simulink model "gm_MATE_HDLsolver_myFirstCircuit"  (R2024b)
settings: Solver=FixedStepDiscrete  StartTime=0.0  StopTime=0.05  FixedStep=6.02409638554217e-09  MaxStep=100e-6  RelTol=1e-4
PostLoadFcn:
  | Ts=1e-6; nb_sw=3; nb_lc=2;nb_r=1;nb_src=1; nb_out=3; rL=1.2;rC=100;L=1e-3; C=1e-5; LpejoSw=1e-6;h=Ts; MAX_INPUTS=16;
  | MAX_OUTPUTS=16;
  | MAX_SWITCHES=8;
  | MAX_INPUTS=16;
InitFcn:
  | Ts=1e-6; nb_sw=3; nb_lc=2;nb_r=1;nb_src=1; nb_out=3; rL=1.2;rC=100;L=1e-3; C=1e-5; LpejoSw=1e-6;h=Ts; MAX_INPUTS=16;
  | MAX_OUTPUTS=16;
  | MAX_SWITCHES=8;
  | MAX_INPUTS=16;
undefined symbols (not defined in the file or in its folder): MATE_SOC
libraries: fl_lib x31, nesl_utility x13, hdlmdlgenlib x10, simetranss x5, simulink x4, hdlsllib x3, ee_lib x2, eeGeneralControl x1
(part 4 of 8)

== system gm_MATE_HDLsolver_myFirstCircuit/ForFPGA/Dot Product1412 ==
  In1 : Inport
  In2 : Inport  Port=2
  Dot Product1412 : Sum  OutDataTypeStr=single  SampleTime=6.02409638554217e-09
  Dot Product1412_pd1 : Delay  DelayLength=6
  Out1 : Outport
  wires:
  In1/1 -> Dot Product1412/1
  In2/1 -> Dot Product1412/2
  Dot Product1412/1 -> Dot Product1412_pd1/1
  Dot Product1412_pd1/1 -> Out1/1

== system gm_MATE_HDLsolver_myFirstCircuit/ForFPGA/Dot Product1413 ==
  In1 : Inport
  In2 : Inport  Port=2
  Dot Product1413 : Sum  OutDataTypeStr=single  SampleTime=6.02409638554217e-09
  Dot Product1413_pd1 : Delay  DelayLength=6
  Out1 : Outport
  wires:
  In1/1 -> Dot Product1413/1
  In2/1 -> Dot Product1413/2
  Dot Product1413/1 -> Dot Product1413_pd1/1
  Dot Product1413_pd1/1 -> Out1/1

== system gm_MATE_HDLsolver_myFirstCircuit/ForFPGA/Dot Product1414 ==
  In1 : Inport
  In2 : Inport  Port=2
  Dot Product1414 : Sum  OutDataTypeStr=single  SampleTime=6.02409638554217e-09
  Dot Product1414_pd1 : Delay  DelayLength=6
  Out1 : Outport
  wires:
  In1/1 -> Dot Product1414/1
  In2/1 -> Dot Product1414/2
  Dot Product1414/1 -> Dot Product1414_pd1/1
  Dot Product1414_pd1/1 -> Out1/1

== system gm_MATE_HDLsolver_myFirstCircuit/ForFPGA/Dot Product1415 ==
  In1 : Inport
  In2 : Inport  Port=2
  Dot Product1415 : Sum  OutDataTypeStr=single  SampleTime=6.02409638554217e-09
  Dot Product1415_pd1 : Delay  DelayLength=6
  Out1 : Outport
  wires:
  In1/1 -> Dot Product1415/1
  In2/1 -> Dot Product1415/2
  Dot Product1415/1 -> Dot Product1415_pd1/1
  Dot Product1415_pd1/1 -> Out1/1

== system gm_MATE_HDLsolver_myFirstCircuit/ForFPGA/Dot Product142 ==
  In1 : Inport
  In2 : Inport  Port=2
  Dot Product142 : Sum  OutDataTypeStr=single  SampleTime=6.02409638554217e-09
  Dot Product142_pd1 : Delay  DelayLength=6
  Out1 : Outport
  wires:
  In1/1 -> Dot Product142/1
  In2/1 -> Dot Product142/2
  Dot Product142/1 -> Dot Product142_pd1/1
  Dot Product142_pd1/1 -> Out1/1

== system gm_MATE_HDLsolver_myFirstCircuit/ForFPGA/Dot Product143 ==
  In1 : Inport
  In2 : Inport  Port=2
  Dot Product143 : Sum  OutDataTypeStr=single  SampleTime=6.02409638554217e-09
  Dot Product143_pd1 : Delay  DelayLength=6
  Out1 : Outport
  wires:
  In1/1 -> Dot Product143/1
  In2/1 -> Dot Product143/2
  Dot Product143/1 -> Dot Product143_pd1/1
  Dot Product143_pd1/1 -> Out1/1

== system gm_MATE_HDLsolver_myFirstCircuit/ForFPGA/Dot Product144 ==
  In1 : Inport
  In2 : Inport  Port=2
  Dot Product144 : Sum  OutDataTypeStr=single  SampleTime=6.02409638554217e-09
  Dot Product144_pd1 : Delay  DelayLength=6
  Out1 : Outport
  wires:
  In1/1 -> Dot Product144/1
  In2/1 -> Dot Product144/2
  Dot Product144/1 -> Dot Product144_pd1/1
  Dot Product144_pd1/1 -> Out1/1

== system gm_MATE_HDLsolver_myFirstCircuit/ForFPGA/Dot Product145 ==
  In1 : Inport
  In2 : Inport  Port=2
  Dot Product145 : Sum  OutDataTypeStr=single  SampleTime=6.02409638554217e-09
  Dot Product145_pd1 : Delay  DelayLength=6
  Out1 : Outport
  wires:
  In1/1 -> Dot Product145/1
  In2/1 -> Dot Product145/2
  Dot Product145/1 -> Dot Product145_pd1/1
  Dot Product145_pd1/1 -> Out1/1

== system gm_MATE_HDLsolver_myFirstCircuit/ForFPGA/Dot Product146 ==
  In1 : Inport
  In2 : Inport  Port=2
  Dot Product146 : Sum  OutDataTypeStr=single  SampleTime=6.02409638554217e-09
  Dot Product146_pd1 : Delay  DelayLength=6
  Out1 : Outport
  wires:
  In1/1 -> Dot Product146/1
  In2/1 -> Dot Product146/2
  Dot Product146/1 -> Dot Product146_pd1/1
  Dot Product146_pd1/1 -> Out1/1

== system gm_MATE_HDLsolver_myFirstCircuit/ForFPGA/Dot Product147 ==
  In1 : Inport
  In2 : Inport  Port=2
  Dot Product147 : Sum  OutDataTypeStr=single  SampleTime=6.02409638554217e-09
  Dot Product147_pd1 : Delay  DelayLength=6
  Out1 : Outport
  wires:
  In1/1 -> Dot Product147/1
  In2/1 -> Dot Product147/2
  Dot Product147/1 -> Dot Product147_pd1/1
  Dot Product147_pd1/1 -> Out1/1

== system gm_MATE_HDLsolver_myFirstCircuit/ForFPGA/Dot Product148 ==
  In1 : Inport
  In2 : Inport  Port=2
  Dot Product148 : Sum  OutDataTypeStr=single  SampleTime=6.02409638554217e-09
  Dot Product148_pd1 : Delay  DelayLength=6
  Out1 : Outport
  wires:
  In1/1 -> Dot Product148/1
  In2/1 -> Dot Product148/2
  Dot Product148/1 -> Dot Product148_pd1/1
  Dot Product148_pd1/1 -> Out1/1

== system gm_MATE_HDLsolver_myFirstCircuit/ForFPGA/Dot Product149 ==
  In1 : Inport
  In2 : Inport  Port=2
  Dot Product149 : Sum  OutDataTypeStr=single  SampleTime=6.02409638554217e-09
  Dot Product149_pd1 : Delay  DelayLength=6
  Out1 : Outport
  wires:
  In1/1 -> Dot Product149/1
  In2/1 -> Dot Product149/2
  Dot Product149/1 -> Dot Product149_pd1/1
  Dot Product149_pd1/1 -> Out1/1

== system gm_MATE_HDLsolver_myFirstCircuit/ForFPGA/Dot Product15 ==
  In1 : Inport
  In2 : Inport  Port=2
  Dot Product15 : Sum  OutDataTypeStr=single  SampleTime=6.02409638554217e-09
  Dot Product15_pd1 : Delay  DelayLength=6
  Out1 : Outport
  wires:
  In1/1 -> Dot Product15/1
  In2/1 -> Dot Product15/2
  Dot Product15/1 -> Dot Product15_pd1/1
  Dot Product15_pd1/1 -> Out1/1

== system gm_MATE_HDLsolver_myFirstCircuit/ForFPGA/Dot Product151 ==
  In1 : Inport
  In2 : Inport  Port=2
  Dot Product151 : Sum  OutDataTypeStr=single  SampleTime=6.02409638554217e-09
  Dot Product151_pd1 : Delay  DelayLength=6
  Out1 : Outport
  wires:
  In1/1 -> Dot Product151/1
  In2/1 -> Dot Product151/2
  Dot Product151/1 -> Dot Product151_pd1/1
  Dot Product151_pd1/1 -> Out1/1

== system gm_MATE_HDLsolver_myFirstCircuit/ForFPGA/Dot Product1510 ==
  In1 : Inport
  In2 : Inport  Port=2
  Dot Product1510 : Sum  OutDataTypeStr=single  SampleTime=6.02409638554217e-09
  Dot Product1510_pd1 : Delay  DelayLength=6
  Out1 : Outport
  wires:
  In1/1 -> Dot Product1510/1
  In2/1 -> Dot Product1510/2
  Dot Product1510/1 -> Dot Product1510_pd1/1
  Dot Product1510_pd1/1 -> Out1/1

== system gm_MATE_HDLsolver_myFirstCircuit/ForFPGA/Dot Product1511 ==
  In1 : Inport
  In2 : Inport  Port=2
  Dot Product1511 : Sum  OutDataTypeStr=single  SampleTime=6.02409638554217e-09
  Dot Product1511_pd1 : Delay  DelayLength=6
  Out1 : Outport
  wires:
  In1/1 -> Dot Product1511/1
  In2/1 -> Dot Product1511/2
  Dot Product1511/1 -> Dot Product1511_pd1/1
  Dot Product1511_pd1/1 -> Out1/1

== system gm_MATE_HDLsolver_myFirstCircuit/ForFPGA/Dot Product1512 ==
  In1 : Inport
  In2 : Inport  Port=2
  Dot Product1512 : Sum  OutDataTypeStr=single  SampleTime=6.02409638554217e-09
  Dot Product1512_pd1 : Delay  DelayLength=6
  Out1 : Outport
  wires:
  In1/1 -> Dot Product1512/1
  In2/1 -> Dot Product1512/2
  Dot Product1512/1 -> Dot Product1512_pd1/1
  Dot Product1512_pd1/1 -> Out1/1

== system gm_MATE_HDLsolver_myFirstCircuit/ForFPGA/Dot Product1513 ==
  In1 : Inport
  In2 : Inport  Port=2
  Dot Product1513 : Sum  OutDataTypeStr=single  SampleTime=6.02409638554217e-09
  Dot Product1513_pd1 : Delay  DelayLength=6
  Out1 : Outport
  wires:
  In1/1 -> Dot Product1513/1
  In2/1 -> Dot Product1513/2
  Dot Product1513/1 -> Dot Product1513_pd1/1
  Dot Product1513_pd1/1 -> Out1/1

== system gm_MATE_HDLsolver_myFirstCircuit/ForFPGA/Dot Product1514 ==
  In1 : Inport
  In2 : Inport  Port=2
  Dot Product1514 : Sum  OutDataTypeStr=single  SampleTime=6.02409638554217e-09
  Dot Product1514_pd1 : Delay  DelayLength=6
  Out1 : Outport
  wires:
  In1/1 -> Dot Product1514/1
  In2/1 -> Dot Product1514/2
  Dot Product1514/1 -> Dot Product1514_pd1/1
  Dot Product1514_pd1/1 -> Out1/1

== system gm_MATE_HDLsolver_myFirstCircuit/ForFPGA/Dot Product1515 ==
  In1 : Inport
  In2 : Inport  Port=2
  Dot Product1515 : Sum  OutDataTypeStr=single  SampleTime=6.02409638554217e-09
  Dot Product1515_pd1 : Delay  DelayLength=6
  Out1 : Outport
  wires:
  In1/1 -> Dot Product1515/1
  In2/1 -> Dot Product1515/2
  Dot Product1515/1 -> Dot Product1515_pd1/1
  Dot Product1515_pd1/1 -> Out1/1

== system gm_MATE_HDLsolver_myFirstCircuit/ForFPGA/Dot Product152 ==
  In1 : Inport
  In2 : Inport  Port=2
  Dot Product152 : Sum  OutDataTypeStr=single  SampleTime=6.02409638554217e-09
  Dot Product152_pd1 : Delay  DelayLength=6
  Out1 : Outport
  wires:
  In1/1 -> Dot Product152/1
  In2/1 -> Dot Product152/2
  Dot Product152/1 -> Dot Product152_pd1/1
  Dot Product152_pd1/1 -> Out1/1

== system gm_MATE_HDLsolver_myFirstCircuit/ForFPGA/Dot Product153 ==
  In1 : Inport
  In2 : Inport  Port=2
  Dot Product153 : Sum  OutDataTypeStr=single  SampleTime=6.02409638554217e-09
  Dot Product153_pd1 : Delay  DelayLength=6
  Out1 : Outport
  wires:
  In1/1 -> Dot Product153/1
  In2/1 -> Dot Product153/2
  Dot Product153/1 -> Dot Product153_pd1/1
  Dot Product153_pd1/1 -> Out1/1

== system gm_MATE_HDLsolver_myFirstCircuit/ForFPGA/Dot Product154 ==
  In1 : Inport
  In2 : Inport  Port=2
  Dot Product154 : Sum  OutDataTypeStr=single  SampleTime=6.02409638554217e-09
  Dot Product154_pd1 : Delay  DelayLength=6
  Out1 : Outport
  wires:
  In1/1 -> Dot Product154/1
  In2/1 -> Dot Product154/2
  Dot Product154/1 -> Dot Product154_pd1/1
  Dot Product154_pd1/1 -> Out1/1

== system gm_MATE_HDLsolver_myFirstCircuit/ForFPGA/Dot Product155 ==
  In1 : Inport
  In2 : Inport  Port=2
  Dot Product155 : Sum  OutDataTypeStr=single  SampleTime=6.02409638554217e-09
  Dot Product155_pd1 : Delay  DelayLength=6
  Out1 : Outport
  wires:
  In1/1 -> Dot Product155/1
  In2/1 -> Dot Product155/2
  Dot Product155/1 -> Dot Product155_pd1/1
  Dot Product155_pd1/1 -> Out1/1

== system gm_MATE_HDLsolver_myFirstCircuit/ForFPGA/Dot Product156 ==
  In1 : Inport
  In2 : Inport  Port=2
  Dot Product156 : Sum  OutDataTypeStr=single  SampleTime=6.02409638554217e-09
  Dot Product156_pd1 : Delay  DelayLength=6
  Out1 : Outport
  wires:
  In1/1 -> Dot Product156/1
  In2/1 -> Dot Product156/2
  Dot Product156/1 -> Dot Product156_pd1/1
  Dot Product156_pd1/1 -> Out1/1

== system gm_MATE_HDLsolver_myFirstCircuit/ForFPGA/Dot Product157 ==
  In1 : Inport
  In2 : Inport  Port=2
  Dot Product157 : Sum  OutDataTypeStr=single  SampleTime=6.02409638554217e-09
  Dot Product157_pd1 : Delay  DelayLength=6
  Out1 : Outport
  wires:
  In1/1 -> Dot Product157/1
  In2/1 -> Dot Product157/2
  Dot Product157/1 -> Dot Product157_pd1/1
  Dot Product157_pd1/1 -> Out1/1

== system gm_MATE_HDLsolver_myFirstCircuit/ForFPGA/Dot Product158 ==
  In1 : Inport
  In2 : Inport  Port=2
  Dot Product158 : Sum  OutDataTypeStr=single  SampleTime=6.02409638554217e-09
  Dot Product158_pd1 : Delay  DelayLength=6
  Out1 : Outport
  wires:
  In1/1 -> Dot Product158/1
  In2/1 -> Dot Product158/2
  Dot Product158/1 -> Dot Product158_pd1/1
  Dot Product158_pd1/1 -> Out1/1

== system gm_MATE_HDLsolver_myFirstCircuit/ForFPGA/Dot Product159 ==
  In1 : Inport
  In2 : Inport  Port=2
  Dot Product159 : Sum  OutDataTypeStr=single  SampleTime=6.02409638554217e-09
  Dot Product159_pd1 : Delay  DelayLength=6
  Out1 : Outport
  wires:
  In1/1 -> Dot Product159/1
  In2/1 -> Dot Product159/2
  Dot Product159/1 -> Dot Product159_pd1/1
  Dot Product159_pd1/1 -> Out1/1

== system gm_MATE_HDLsolver_myFirstCircuit/ForFPGA/Dot Product16 ==
  In1 : Inport
  In2 : Inport  Port=2
  Dot Product16 : Sum  OutDataTypeStr=single  SampleTime=6.02409638554217e-09
  Dot Product16_pd1 : Delay  DelayLength=6
  Out1 : Outport
  wires:
  In1/1 -> Dot Product16/1
  In2/1 -> Dot Product16/2
  Dot Product16/1 -> Dot Product16_pd1/1
  Dot Product16_pd1/1 -> Out1/1

== system gm_MATE_HDLsolver_myFirstCircuit/ForFPGA/Dot Product17 ==
  In1 : Inport
  In2 : Inport  Port=2
  Dot Product17 : Sum  OutDataTypeStr=single  SampleTime=6.02409638554217e-09
  Dot Product17_pd1 : Delay  DelayLength=6
  Out1 : Outport
  wires:
  In1/1 -> Dot Product17/1
  In2/1 -> Dot Product17/2
  Dot Product17/1 -> Dot Product17_pd1/1
  Dot Product17_pd1/1 -> Out1/1

== system gm_MATE_HDLsolver_myFirstCircuit/ForFPGA/Dot Product18 ==
  In1 : Inport
  In2 : Inport  Port=2
  Dot Product18 : Sum  OutDataTypeStr=single  SampleTime=6.02409638554217e-09
  Dot Product18_pd1 : Delay  DelayLength=6
  Out1 : Outport
  wires:
  In1/1 -> Dot Product18/1
  In2/1 -> Dot Product18/2
  Dot Product18/1 -> Dot Product18_pd1/1
  Dot Product18_pd1/1 -> Out1/1

== system gm_MATE_HDLsolver_myFirstCircuit/ForFPGA/Dot Product19 ==
  In1 : Inport
  In2 : Inport  Port=2
  Dot Product19 : Sum  OutDataTypeStr=single  SampleTime=6.02409638554217e-09
  Dot Product19_pd1 : Delay  DelayLength=6
  Out1 : Outport
  wires:
  In1/1 -> Dot Product19/1
  In2/1 -> Dot Product19/2
  Dot Product19/1 -> Dot Product19_pd1/1
  Dot Product19_pd1/1 -> Out1/1

== system gm_MATE_HDLsolver_myFirstCircuit/ForFPGA/Dot Product2 ==
  In1 : Inport
  In2 : Inport  Port=2
  Dot Product2 : Sum  OutDataTypeStr=single  SampleTime=6.02409638554217e-09
  Dot Product2_pd1 : Delay  DelayLength=6
  Out1 : Outport
  wires:
  In1/1 -> Dot Product2/1
  In2/1 -> Dot Product2/2
  Dot Product2/1 -> Dot Product2_pd1/1
  Dot Product2_pd1/1 -> Out1/1

== system gm_MATE_HDLsolver_myFirstCircuit/ForFPGA/Dot Product21 ==
  In1 : Inport
  In2 : Inport  Port=2
  Dot Product21 : Sum  OutDataTypeStr=single  SampleTime=6.02409638554217e-09
  Dot Product21_pd1 : Delay  DelayLength=6
  Out1 : Outport
  wires:
  In1/1 -> Dot Product21/1
  In2/1 -> Dot Product21/2
  Dot Product21/1 -> Dot Product21_pd1/1
  Dot Product21_pd1/1 -> Out1/1

== system gm_MATE_HDLsolver_myFirstCircuit/ForFPGA/Dot Product210 ==
  In1 : Inport
  In2 : Inport  Port=2
  Dot Product210 : Sum  OutDataTypeStr=single  SampleTime=6.02409638554217e-09
  Dot Product210_pd1 : Delay  DelayLength=6
  Out1 : Outport
  wires:
  In1/1 -> Dot Product210/1
  In2/1 -> Dot Product210/2
  Dot Product210/1 -> Dot Product210_pd1/1
  Dot Product210_pd1/1 -> Out1/1

== system gm_MATE_HDLsolver_myFirstCircuit/ForFPGA/Dot Product211 ==
  In1 : Inport
  In2 : Inport  Port=2
  Dot Product211 : Sum  OutDataTypeStr=single  SampleTime=6.02409638554217e-09
  Dot Product211_pd1 : Delay  DelayLength=6
  Out1 : Outport
  wires:
  In1/1 -> Dot Product211/1
  In2/1 -> Dot Product211/2
  Dot Product211/1 -> Dot Product211_pd1/1
  Dot Product211_pd1/1 -> Out1/1

== system gm_MATE_HDLsolver_myFirstCircuit/ForFPGA/Dot Product212 ==
  In1 : Inport
  In2 : Inport  Port=2
  Dot Product212 : Sum  OutDataTypeStr=single  SampleTime=6.02409638554217e-09
  Dot Product212_pd1 : Delay  DelayLength=6
  Out1 : Outport
  wires:
  In1/1 -> Dot Product212/1
  In2/1 -> Dot Product212/2
  Dot Product212/1 -> Dot Product212_pd1/1
  Dot Product212_pd1/1 -> Out1/1

== system gm_MATE_HDLsolver_myFirstCircuit/ForFPGA/Dot Product213 ==
  In1 : Inport
  In2 : Inport  Port=2
  Dot Product213 : Sum  OutDataTypeStr=single  SampleTime=6.02409638554217e-09
  Dot Product213_pd1 : Delay  DelayLength=6
  Out1 : Outport
  wires:
  In1/1 -> Dot Product213/1
  In2/1 -> Dot Product213/2
  Dot Product213/1 -> Dot Product213_pd1/1
  Dot Product213_pd1/1 -> Out1/1

== system gm_MATE_HDLsolver_myFirstCircuit/ForFPGA/Dot Product214 ==
  In1 : Inport
  In2 : Inport  Port=2
  Dot Product214 : Sum  OutDataTypeStr=single  SampleTime=6.02409638554217e-09
  Dot Product214_pd1 : Delay  DelayLength=6
  Out1 : Outport
  wires:
  In1/1 -> Dot Product214/1
  In2/1 -> Dot Product214/2
  Dot Product214/1 -> Dot Product214_pd1/1
  Dot Product214_pd1/1 -> Out1/1

== system gm_MATE_HDLsolver_myFirstCircuit/ForFPGA/Dot Product215 ==
  In1 : Inport
  In2 : Inport  Port=2
  Dot Product215 : Sum  OutDataTypeStr=single  SampleTime=6.02409638554217e-09
  Dot Product215_pd1 : Delay  DelayLength=6
  Out1 : Outport
  wires:
  In1/1 -> Dot Product215/1
  In2/1 -> Dot Product215/2
  Dot Product215/1 -> Dot Product215_pd1/1
  Dot Product215_pd1/1 -> Out1/1

== system gm_MATE_HDLsolver_myFirstCircuit/ForFPGA/Dot Product22 ==
  In1 : Inport
  In2 : Inport  Port=2
  Dot Product22 : Sum  OutDataTypeStr=single  SampleTime=6.02409638554217e-09
  Dot Product22_pd1 : Delay  DelayLength=6
  Out1 : Outport
  wires:
  In1/1 -> Dot Product22/1
  In2/1 -> Dot Product22/2
  Dot Product22/1 -> Dot Product22_pd1/1
  Dot Product22_pd1/1 -> Out1/1

== system gm_MATE_HDLsolver_myFirstCircuit/ForFPGA/Dot Product23 ==
  In1 : Inport
  In2 : Inport  Port=2
  Dot Product23 : Sum  OutDataTypeStr=single  SampleTime=6.02409638554217e-09
  Dot Product23_pd1 : Delay  DelayLength=6
  Out1 : Outport
  wires:
  In1/1 -> Dot Product23/1
  In2/1 -> Dot Product23/2
  Dot Product23/1 -> Dot Product23_pd1/1
  Dot Product23_pd1/1 -> Out1/1

== system gm_MATE_HDLsolver_myFirstCircuit/ForFPGA/Dot Product24 ==
  In1 : Inport
  In2 : Inport  Port=2
  Dot Product24 : Sum  OutDataTypeStr=single  SampleTime=6.02409638554217e-09
  Dot Product24_pd1 : Delay  DelayLength=6
  Out1 : Outport
  wires:
  In1/1 -> Dot Product24/1
  In2/1 -> Dot Product24/2
  Dot Product24/1 -> Dot Product24_pd1/1
  Dot Product24_pd1/1 -> Out1/1

== system gm_MATE_HDLsolver_myFirstCircuit/ForFPGA/Dot Product25 ==
  In1 : Inport
  In2 : Inport  Port=2
  Dot Product25 : Sum  OutDataTypeStr=single  SampleTime=6.02409638554217e-09
  Dot Product25_pd1 : Delay  DelayLength=6
  Out1 : Outport
  wires:
  In1/1 -> Dot Product25/1
  In2/1 -> Dot Product25/2
  Dot Product25/1 -> Dot Product25_pd1/1
  Dot Product25_pd1/1 -> Out1/1

== system gm_MATE_HDLsolver_myFirstCircuit/ForFPGA/Dot Product26 ==
  In1 : Inport
  In2 : Inport  Port=2
  Dot Product26 : Sum  OutDataTypeStr=single  SampleTime=6.02409638554217e-09
  Dot Product26_pd1 : Delay  DelayLength=6
  Out1 : Outport
  wires:
  In1/1 -> Dot Product26/1
  In2/1 -> Dot Product26/2
  Dot Product26/1 -> Dot Product26_pd1/1
  Dot Product26_pd1/1 -> Out1/1

== system gm_MATE_HDLsolver_myFirstCircuit/ForFPGA/Dot Product27 ==
  In1 : Inport
  In2 : Inport  Port=2
  Dot Product27 : Sum  OutDataTypeStr=single  SampleTime=6.02409638554217e-09
  Dot Product27_pd1 : Delay  DelayLength=6
  Out1 : Outport
  wires:
  In1/1 -> Dot Product27/1
  In2/1 -> Dot Product27/2
  Dot Product27/1 -> Dot Product27_pd1/1
  Dot Product27_pd1/1 -> Out1/1

== system gm_MATE_HDLsolver_myFirstCircuit/ForFPGA/Dot Product28 ==
  In1 : Inport
  In2 : Inport  Port=2
  Dot Product28 : Sum  OutDataTypeStr=single  SampleTime=6.02409638554217e-09
  Dot Product28_pd1 : Delay  DelayLength=6
  Out1 : Outport
  wires:
  In1/1 -> Dot Product28/1
  In2/1 -> Dot Product28/2
  Dot Product28/1 -> Dot Product28_pd1/1
  Dot Product28_pd1/1 -> Out1/1

== system gm_MATE_HDLsolver_myFirstCircuit/ForFPGA/Dot Product29 ==
  In1 : Inport
  In2 : Inport  Port=2
  Dot Product29 : Sum  OutDataTypeStr=single  SampleTime=6.02409638554217e-09
  Dot Product29_pd1 : Delay  DelayLength=6
  Out1 : Outport
  wires:
  In1/1 -> Dot Product29/1
  In2/1 -> Dot Product29/2
  Dot Product29/1 -> Dot Product29_pd1/1
  Dot Product29_pd1/1 -> Out1/1

== system gm_MATE_HDLsolver_myFirstCircuit/ForFPGA/Dot Product3 ==
  In1 : Inport
  In2 : Inport  Port=2
  Dot Product3 : Sum  OutDataTypeStr=single  SampleTime=6.02409638554217e-09
  Dot Product3_pd1 : Delay  DelayLength=6
  Out1 : Outport
  wires:
  In1/1 -> Dot Product3/1
  In2/1 -> Dot Product3/2
  Dot Product3/1 -> Dot Product3_pd1/1
  Dot Product3_pd1/1 -> Out1/1

== system gm_MATE_HDLsolver_myFirstCircuit/ForFPGA/Dot Product31 ==
  In1 : Inport
  In2 : Inport  Port=2
  Dot Product31 : Sum  OutDataTypeStr=single  SampleTime=6.02409638554217e-09
  Dot Product31_pd1 : Delay  DelayLength=6
  Out1 : Outport
  wires:
  In1/1 -> Dot Product31/1
  In2/1 -> Dot Product31/2
  Dot Product31/1 -> Dot Product31_pd1/1
  Dot Product31_pd1/1 -> Out1/1

== system gm_MATE_HDLsolver_myFirstCircuit/ForFPGA/Dot Product310 ==
  In1 : Inport
  In2 : Inport  Port=2
  Dot Product310 : Sum  OutDataTypeStr=single  SampleTime=6.02409638554217e-09
  Dot Product310_pd1 : Delay  DelayLength=6
  Out1 : Outport
  wires:
  In1/1 -> Dot Product310/1
  In2/1 -> Dot Product310/2
  Dot Product310/1 -> Dot Product310_pd1/1
  Dot Product310_pd1/1 -> Out1/1

== system gm_MATE_HDLsolver_myFirstCircuit/ForFPGA/Dot Product311 ==
  In1 : Inport
  In2 : Inport  Port=2
  Dot Product311 : Sum  OutDataTypeStr=single  SampleTime=6.02409638554217e-09
  Dot Product311_pd1 : Delay  DelayLength=6
  Out1 : Outport
  wires:
  In1/1 -> Dot Product311/1
  In2/1 -> Dot Product311/2
  Dot Product311/1 -> Dot Product311_pd1/1
  Dot Product311_pd1/1 -> Out1/1

== system gm_MATE_HDLsolver_myFirstCircuit/ForFPGA/Dot Product312 ==
  In1 : Inport
  In2 : Inport  Port=2
  Dot Product312 : Sum  OutDataTypeStr=single  SampleTime=6.02409638554217e-09
  Dot Product312_pd1 : Delay  DelayLength=6
  Out1 : Outport
  wires:
  In1/1 -> Dot Product312/1
  In2/1 -> Dot Product312/2
  Dot Product312/1 -> Dot Product312_pd1/1
  Dot Product312_pd1/1 -> Out1/1

== system gm_MATE_HDLsolver_myFirstCircuit/ForFPGA/Dot Product313 ==
  In1 : Inport
  In2 : Inport  Port=2
  Dot Product313 : Sum  OutDataTypeStr=single  SampleTime=6.02409638554217e-09
  Dot Product313_pd1 : Delay  DelayLength=6
  Out1 : Outport
  wires:
  In1/1 -> Dot Product313/1
  In2/1 -> Dot Product313/2
  Dot Product313/1 -> Dot Product313_pd1/1
  Dot Product313_pd1/1 -> Out1/1

== system gm_MATE_HDLsolver_myFirstCircuit/ForFPGA/Dot Product314 ==
  In1 : Inport
  In2 : Inport  Port=2
  Dot Product314 : Sum  OutDataTypeStr=single  SampleTime=6.02409638554217e-09
  Dot Product314_pd1 : Delay  DelayLength=6
  Out1 : Outport
  wires:
  In1/1 -> Dot Product314/1
  In2/1 -> Dot Product314/2
  Dot Product314/1 -> Dot Product314_pd1/1
  Dot Product314_pd1/1 -> Out1/1

== system gm_MATE_HDLsolver_myFirstCircuit/ForFPGA/Dot Product315 ==
  In1 : Inport
  In2 : Inport  Port=2
  Dot Product315 : Sum  OutDataTypeStr=single  SampleTime=6.02409638554217e-09
  Dot Product315_pd1 : Delay  DelayLength=6
  Out1 : Outport
  wires:
  In1/1 -> Dot Product315/1
  In2/1 -> Dot Product315/2
  Dot Product315/1 -> Dot Product315_pd1/1
  Dot Product315_pd1/1 -> Out1/1

== system gm_MATE_HDLsolver_myFirstCircuit/ForFPGA/Dot Product32 ==
  In1 : Inport
  In2 : Inport  Port=2
  Dot Product32 : Sum  OutDataTypeStr=single  SampleTime=6.02409638554217e-09
  Dot Product32_pd1 : Delay  DelayLength=6
  Out1 : Outport
  wires:
  In1/1 -> Dot Product32/1
  In2/1 -> Dot Product32/2
  Dot Product32/1 -> Dot Product32_pd1/1
  Dot Product32_pd1/1 -> Out1/1

== system gm_MATE_HDLsolver_myFirstCircuit/ForFPGA/Dot Product33 ==
  In1 : Inport
  In2 : Inport  Port=2
  Dot Product33 : Sum  OutDataTypeStr=single  SampleTime=6.02409638554217e-09
  Dot Product33_pd1 : Delay  DelayLength=6
  Out1 : Outport
  wires:
  In1/1 -> Dot Product33/1
  In2/1 -> Dot Product33/2
  Dot Product33/1 -> Dot Product33_pd1/1
  Dot Product33_pd1/1 -> Out1/1

== system gm_MATE_HDLsolver_myFirstCircuit/ForFPGA/Dot Product34 ==
  In1 : Inport
  In2 : Inport  Port=2
  Dot Product34 : Sum  OutDataTypeStr=single  SampleTime=6.02409638554217e-09
  Dot Product34_pd1 : Delay  DelayLength=6
  Out1 : Outport
  wires:
  In1/1 -> Dot Product34/1
  In2/1 -> Dot Product34/2
  Dot Product34/1 -> Dot Product34_pd1/1
  Dot Product34_pd1/1 -> Out1/1

== system gm_MATE_HDLsolver_myFirstCircuit/ForFPGA/Dot Product35 ==
  In1 : Inport
  In2 : Inport  Port=2
  Dot Product35 : Sum  OutDataTypeStr=single  SampleTime=6.02409638554217e-09
  Dot Product35_pd1 : Delay  DelayLength=6
  Out1 : Outport
  wires:
  In1/1 -> Dot Product35/1
  In2/1 -> Dot Product35/2
  Dot Product35/1 -> Dot Product35_pd1/1
  Dot Product35_pd1/1 -> Out1/1

== system gm_MATE_HDLsolver_myFirstCircuit/ForFPGA/Dot Product36 ==
  In1 : Inport
  In2 : Inport  Port=2
  Dot Product36 : Sum  OutDataTypeStr=single  SampleTime=6.02409638554217e-09
  Dot Product36_pd1 : Delay  DelayLength=6
  Out1 : Outport
  wires:
  In1/1 -> Dot Product36/1
  In2/1 -> Dot Product36/2
  Dot Product36/1 -> Dot Product36_pd1/1
  Dot Product36_pd1/1 -> Out1/1

== system gm_MATE_HDLsolver_myFirstCircuit/ForFPGA/Dot Product37 ==
  In1 : Inport
  In2 : Inport  Port=2
  Dot Product37 : Sum  OutDataTypeStr=single  SampleTime=6.02409638554217e-09
  Dot Product37_pd1 : Delay  DelayLength=6
  Out1 : Outport
  wires:
  In1/1 -> Dot Product37/1
  In2/1 -> Dot Product37/2
  Dot Product37/1 -> Dot Product37_pd1/1
  Dot Product37_pd1/1 -> Out1/1

== system gm_MATE_HDLsolver_myFirstCircuit/ForFPGA/Dot Product38 ==
  In1 : Inport
  In2 : Inport  Port=2
  Dot Product38 : Sum  OutDataTypeStr=single  SampleTime=6.02409638554217e-09
  Dot Product38_pd1 : Delay  DelayLength=6
  Out1 : Outport
  wires:
  In1/1 -> Dot Product38/1
  In2/1 -> Dot Product38/2
  Dot Product38/1 -> Dot Product38_pd1/1
  Dot Product38_pd1/1 -> Out1/1

== system gm_MATE_HDLsolver_myFirstCircuit/ForFPGA/Dot Product39 ==
  In1 : Inport
  In2 : Inport  Port=2
  Dot Product39 : Sum  OutDataTypeStr=single  SampleTime=6.02409638554217e-09
  Dot Product39_pd1 : Delay  DelayLength=6
  Out1 : Outport
  wires:
  In1/1 -> Dot Product39/1
  In2/1 -> Dot Product39/2
  Dot Product39/1 -> Dot Product39_pd1/1
  Dot Product39_pd1/1 -> Out1/1

== system gm_MATE_HDLsolver_myFirstCircuit/ForFPGA/Dot Product4 ==
  In1 : Inport
  In2 : Inport  Port=2
  Dot Product4 : Sum  OutDataTypeStr=single  SampleTime=6.02409638554217e-09
  Dot Product4_pd1 : Delay  DelayLength=6
  Out1 : Outport
  wires:
  In1/1 -> Dot Product4/1
  In2/1 -> Dot Product4/2
  Dot Product4/1 -> Dot Product4_pd1/1
  Dot Product4_pd1/1 -> Out1/1

== system gm_MATE_HDLsolver_myFirstCircuit/ForFPGA/Dot Product41 ==
  In1 : Inport
  In2 : Inport  Port=2
  Dot Product41 : Sum  OutDataTypeStr=single  SampleTime=6.02409638554217e-09
  Dot Product41_pd1 : Delay  DelayLength=6
  Out1 : Outport
  wires:
  In1/1 -> Dot Product41/1
  In2/1 -> Dot Product41/2
  Dot Product41/1 -> Dot Product41_pd1/1
  Dot Product41_pd1/1 -> Out1/1

== system gm_MATE_HDLsolver_myFirstCircuit/ForFPGA/Dot Product410 ==
  In1 : Inport
  In2 : Inport  Port=2
  Dot Product410 : Sum  OutDataTypeStr=single  SampleTime=6.02409638554217e-09
  Dot Product410_pd1 : Delay  DelayLength=6
  Out1 : Outport
  wires:
  In1/1 -> Dot Product410/1
  In2/1 -> Dot Product410/2
  Dot Product410/1 -> Dot Product410_pd1/1
  Dot Product410_pd1/1 -> Out1/1

== system gm_MATE_HDLsolver_myFirstCircuit/ForFPGA/Dot Product411 ==
  In1 : Inport
  In2 : Inport  Port=2
  Dot Product411 : Sum  OutDataTypeStr=single  SampleTime=6.02409638554217e-09
  Dot Product411_pd1 : Delay  DelayLength=6
  Out1 : Outport
  wires:
  In1/1 -> Dot Product411/1
  In2/1 -> Dot Product411/2
  Dot Product411/1 -> Dot Product411_pd1/1
  Dot Product411_pd1/1 -> Out1/1

== system gm_MATE_HDLsolver_myFirstCircuit/ForFPGA/Dot Product412 ==
  In1 : Inport
  In2 : Inport  Port=2
  Dot Product412 : Sum  OutDataTypeStr=single  SampleTime=6.02409638554217e-09
  Dot Product412_pd1 : Delay  DelayLength=6
  Out1 : Outport
  wires:
  In1/1 -> Dot Product412/1
  In2/1 -> Dot Product412/2
  Dot Product412/1 -> Dot Product412_pd1/1
  Dot Product412_pd1/1 -> Out1/1

== system gm_MATE_HDLsolver_myFirstCircuit/ForFPGA/Dot Product413 ==
  In1 : Inport
  In2 : Inport  Port=2
  Dot Product413 : Sum  OutDataTypeStr=single  SampleTime=6.02409638554217e-09
  Dot Product413_pd1 : Delay  DelayLength=6
  Out1 : Outport
  wires:
  In1/1 -> Dot Product413/1
  In2/1 -> Dot Product413/2
  Dot Product413/1 -> Dot Product413_pd1/1
  Dot Product413_pd1/1 -> Out1/1

== system gm_MATE_HDLsolver_myFirstCircuit/ForFPGA/Dot Product414 ==
  In1 : Inport
  In2 : Inport  Port=2
  Dot Product414 : Sum  OutDataTypeStr=single  SampleTime=6.02409638554217e-09
  Dot Product414_pd1 : Delay  DelayLength=6
  Out1 : Outport
  wires:
  In1/1 -> Dot Product414/1
  In2/1 -> Dot Product414/2
  Dot Product414/1 -> Dot Product414_pd1/1
  Dot Product414_pd1/1 -> Out1/1

== system gm_MATE_HDLsolver_myFirstCircuit/ForFPGA/Dot Product415 ==
  In1 : Inport
  In2 : Inport  Port=2
  Dot Product415 : Sum  OutDataTypeStr=single  SampleTime=6.02409638554217e-09
  Dot Product415_pd1 : Delay  DelayLength=6
  Out1 : Outport
  wires:
  In1/1 -> Dot Product415/1
  In2/1 -> Dot Product415/2
  Dot Product415/1 -> Dot Product415_pd1/1
  Dot Product415_pd1/1 -> Out1/1

== system gm_MATE_HDLsolver_myFirstCircuit/ForFPGA/Dot Product42 ==
  In1 : Inport
  In2 : Inport  Port=2
  Dot Product42 : Sum  OutDataTypeStr=single  SampleTime=6.02409638554217e-09
  Dot Product42_pd1 : Delay  DelayLength=6
  Out1 : Outport
  wires:
  In1/1 -> Dot Product42/1
  In2/1 -> Dot Product42/2
  Dot Product42/1 -> Dot Product42_pd1/1
  Dot Product42_pd1/1 -> Out1/1

== system gm_MATE_HDLsolver_myFirstCircuit/ForFPGA/Dot Product43 ==
  In1 : Inport
  In2 : Inport  Port=2
  Dot Product43 : Sum  OutDataTypeStr=single  SampleTime=6.02409638554217e-09
  Dot Product43_pd1 : Delay  DelayLength=6
  Out1 : Outport
  wires:
  In1/1 -> Dot Product43/1
  In2/1 -> Dot Product43/2
  Dot Product43/1 -> Dot Product43_pd1/1
  Dot Product43_pd1/1 -> Out1/1

== system gm_MATE_HDLsolver_myFirstCircuit/ForFPGA/Dot Product44 ==
  In1 : Inport
  In2 : Inport  Port=2
  Dot Product44 : Sum  OutDataTypeStr=single  SampleTime=6.02409638554217e-09
  Dot Product44_pd1 : Delay  DelayLength=6
  Out1 : Outport
  wires:
  In1/1 -> Dot Product44/1
  In2/1 -> Dot Product44/2
  Dot Product44/1 -> Dot Product44_pd1/1
  Dot Product44_pd1/1 -> Out1/1

== system gm_MATE_HDLsolver_myFirstCircuit/ForFPGA/Dot Product45 ==
  In1 : Inport
  In2 : Inport  Port=2
  Dot Product45 : Sum  OutDataTypeStr=single  SampleTime=6.02409638554217e-09
  Dot Product45_pd1 : Delay  DelayLength=6
  Out1 : Outport
  wires:
  In1/1 -> Dot Product45/1
  In2/1 -> Dot Product45/2
  Dot Product45/1 -> Dot Product45_pd1/1
  Dot Product45_pd1/1 -> Out1/1

== system gm_MATE_HDLsolver_myFirstCircuit/ForFPGA/Dot Product46 ==
  In1 : Inport
  In2 : Inport  Port=2
  Dot Product46 : Sum  OutDataTypeStr=single  SampleTime=6.02409638554217e-09
  Dot Product46_pd1 : Delay  DelayLength=6
  Out1 : Outport
  wires:
  In1/1 -> Dot Product46/1
  In2/1 -> Dot Product46/2
  Dot Product46/1 -> Dot Product46_pd1/1
  Dot Product46_pd1/1 -> Out1/1

== system gm_MATE_HDLsolver_myFirstCircuit/ForFPGA/Dot Product47 ==
  In1 : Inport
  In2 : Inport  Port=2
  Dot Product47 : Sum  OutDataTypeStr=single  SampleTime=6.02409638554217e-09
  Dot Product47_pd1 : Delay  DelayLength=6
  Out1 : Outport
  wires:
  In1/1 -> Dot Product47/1
  In2/1 -> Dot Product47/2
  Dot Product47/1 -> Dot Product47_pd1/1
  Dot Product47_pd1/1 -> Out1/1

== system gm_MATE_HDLsolver_myFirstCircuit/ForFPGA/Dot Product48 ==
  In1 : Inport
  In2 : Inport  Port=2
  Dot Product48 : Sum  OutDataTypeStr=single  SampleTime=6.02409638554217e-09
  Dot Product48_pd1 : Delay  DelayLength=6
  Out1 : Outport
  wires:
  In1/1 -> Dot Product48/1
  In2/1 -> Dot Product48/2
  Dot Product48/1 -> Dot Product48_pd1/1
  Dot Product48_pd1/1 -> Out1/1

== system gm_MATE_HDLsolver_myFirstCircuit/ForFPGA/Dot Product49 ==
  In1 : Inport
  In2 : Inport  Port=2
  Dot Product49 : Sum  OutDataTypeStr=single  SampleTime=6.02409638554217e-09
  Dot Product49_pd1 : Delay  DelayLength=6
  Out1 : Outport
  wires:
  In1/1 -> Dot Product49/1
  In2/1 -> Dot Product49/2
  Dot Product49/1 -> Dot Product49_pd1/1
  Dot Product49_pd1/1 -> Out1/1

== system gm_MATE_HDLsolver_myFirstCircuit/ForFPGA/Dot Product5 ==
  In1 : Inport
  In2 : Inport  Port=2
  Dot Product5 : Sum  OutDataTypeStr=single  SampleTime=6.02409638554217e-09
  Dot Product5_pd1 : Delay  DelayLength=6
  Out1 : Outport
  wires:
  In1/1 -> Dot Product5/1
  In2/1 -> Dot Product5/2
  Dot Product5/1 -> Dot Product5_pd1/1
  Dot Product5_pd1/1 -> Out1/1

== system gm_MATE_HDLsolver_myFirstCircuit/ForFPGA/Dot Product51 ==
  In1 : Inport
  In2 : Inport  Port=2
  Dot Product51 : Sum  OutDataTypeStr=single  SampleTime=6.02409638554217e-09
  Dot Product51_pd1 : Delay  DelayLength=6
  Out1 : Outport
  wires:
  In1/1 -> Dot Product51/1
  In2/1 -> Dot Product51/2
  Dot Product51/1 -> Dot Product51_pd1/1
  Dot Product51_pd1/1 -> Out1/1

== system gm_MATE_HDLsolver_myFirstCircuit/ForFPGA/Dot Product510 ==
  In1 : Inport
  In2 : Inport  Port=2
  Dot Product510 : Sum  OutDataTypeStr=single  SampleTime=6.02409638554217e-09
  Dot Product510_pd1 : Delay  DelayLength=6
  Out1 : Outport
  wires:
  In1/1 -> Dot Product510/1
  In2/1 -> Dot Product510/2
  Dot Product510/1 -> Dot Product510_pd1/1
  Dot Product510_pd1/1 -> Out1/1

== system gm_MATE_HDLsolver_myFirstCircuit/ForFPGA/Dot Product511 ==
  In1 : Inport
  In2 : Inport  Port=2
  Dot Product511 : Sum  OutDataTypeStr=single  SampleTime=6.02409638554217e-09
  Dot Product511_pd1 : Delay  DelayLength=6
  Out1 : Outport
  wires:
  In1/1 -> Dot Product511/1
  In2/1 -> Dot Product511/2
  Dot Product511/1 -> Dot Product511_pd1/1
  Dot Product511_pd1/1 -> Out1/1

== system gm_MATE_HDLsolver_myFirstCircuit/ForFPGA/Dot Product512 ==
  In1 : Inport
  In2 : Inport  Port=2
  Dot Product512 : Sum  OutDataTypeStr=single  SampleTime=6.02409638554217e-09
  Dot Product512_pd1 : Delay  DelayLength=6
  Out1 : Outport
  wires:
  In1/1 -> Dot Product512/1
  In2/1 -> Dot Product512/2
  Dot Product512/1 -> Dot Product512_pd1/1
  Dot Product512_pd1/1 -> Out1/1

== system gm_MATE_HDLsolver_myFirstCircuit/ForFPGA/Dot Product513 ==
  In1 : Inport
  In2 : Inport  Port=2
  Dot Product513 : Sum  OutDataTypeStr=single  SampleTime=6.02409638554217e-09
  Dot Product513_pd1 : Delay  DelayLength=6
  Out1 : Outport
  wires:
  In1/1 -> Dot Product513/1
  In2/1 -> Dot Product513/2
  Dot Product513/1 -> Dot Product513_pd1/1
  Dot Product513_pd1/1 -> Out1/1

== system gm_MATE_HDLsolver_myFirstCircuit/ForFPGA/Dot Product514 ==
  In1 : Inport
  In2 : Inport  Port=2
  Dot Product514 : Sum  OutDataTypeStr=single  SampleTime=6.02409638554217e-09
  Dot Product514_pd1 : Delay  DelayLength=6
  Out1 : Outport
  wires:
  In1/1 -> Dot Product514/1
  In2/1 -> Dot Product514/2
  Dot Product514/1 -> Dot Product514_pd1/1
  Dot Product514_pd1/1 -> Out1/1

== system gm_MATE_HDLsolver_myFirstCircuit/ForFPGA/Dot Product515 ==
  In1 : Inport
  In2 : Inport  Port=2
  Dot Product515 : Sum  OutDataTypeStr=single  SampleTime=6.02409638554217e-09
  Dot Product515_pd1 : Delay  DelayLength=6
  Out1 : Outport
  wires:
  In1/1 -> Dot Product515/1
  In2/1 -> Dot Product515/2
  Dot Product515/1 -> Dot Product515_pd1/1
  Dot Product515_pd1/1 -> Out1/1

== system gm_MATE_HDLsolver_myFirstCircuit/ForFPGA/Dot Product52 ==
  In1 : Inport
  In2 : Inport  Port=2
  Dot Product52 : Sum  OutDataTypeStr=single  SampleTime=6.02409638554217e-09
  Dot Product52_pd1 : Delay  DelayLength=6
  Out1 : Outport
  wires:
  In1/1 -> Dot Product52/1
  In2/1 -> Dot Product52/2
  Dot Product52/1 -> Dot Product52_pd1/1
  Dot Product52_pd1/1 -> Out1/1

== system gm_MATE_HDLsolver_myFirstCircuit/ForFPGA/Dot Product53 ==
  In1 : Inport
  In2 : Inport  Port=2
  Dot Product53 : Sum  OutDataTypeStr=single  SampleTime=6.02409638554217e-09
  Dot Product53_pd1 : Delay  DelayLength=6
  Out1 : Outport
  wires:
  In1/1 -> Dot Product53/1
  In2/1 -> Dot Product53/2
  Dot Product53/1 -> Dot Product53_pd1/1
  Dot Product53_pd1/1 -> Out1/1

== system gm_MATE_HDLsolver_myFirstCircuit/ForFPGA/Dot Product54 ==
  In1 : Inport
  In2 : Inport  Port=2
  Dot Product54 : Sum  OutDataTypeStr=single  SampleTime=6.02409638554217e-09
  Dot Product54_pd1 : Delay  DelayLength=6
  Out1 : Outport
  wires:
  In1/1 -> Dot Product54/1
  In2/1 -> Dot Product54/2
  Dot Product54/1 -> Dot Product54_pd1/1
  Dot Product54_pd1/1 -> Out1/1

== system gm_MATE_HDLsolver_myFirstCircuit/ForFPGA/Dot Product55 ==
  In1 : Inport
  In2 : Inport  Port=2
  Dot Product55 : Sum  OutDataTypeStr=single  SampleTime=6.02409638554217e-09
  Dot Product55_pd1 : Delay  DelayLength=6
  Out1 : Outport
  wires:
  In1/1 -> Dot Product55/1
  In2/1 -> Dot Product55/2
  Dot Product55/1 -> Dot Product55_pd1/1
  Dot Product55_pd1/1 -> Out1/1

== system gm_MATE_HDLsolver_myFirstCircuit/ForFPGA/Dot Product56 ==
  In1 : Inport
  In2 : Inport  Port=2
  Dot Product56 : Sum  OutDataTypeStr=single  SampleTime=6.02409638554217e-09
  Dot Product56_pd1 : Delay  DelayLength=6
  Out1 : Outport
  wires:
  In1/1 -> Dot Product56/1
  In2/1 -> Dot Product56/2
  Dot Product56/1 -> Dot Product56_pd1/1
  Dot Product56_pd1/1 -> Out1/1

== system gm_MATE_HDLsolver_myFirstCircuit/ForFPGA/Dot Product57 ==
  In1 : Inport
  In2 : Inport  Port=2
  Dot Product57 : Sum  OutDataTypeStr=single  SampleTime=6.02409638554217e-09
  Dot Product57_pd1 : Delay  DelayLength=6
  Out1 : Outport
  wires:
  In1/1 -> Dot Product57/1
  In2/1 -> Dot Product57/2
  Dot Product57/1 -> Dot Product57_pd1/1
  Dot Product57_pd1/1 -> Out1/1

== system gm_MATE_HDLsolver_myFirstCircuit/ForFPGA/Dot Product58 ==
  In1 : Inport
  In2 : Inport  Port=2
  Dot Product58 : Sum  OutDataTypeStr=single  SampleTime=6.02409638554217e-09
  Dot Product58_pd1 : Delay  DelayLength=6
  Out1 : Outport
  wires:
  In1/1 -> Dot Product58/1
  In2/1 -> Dot Product58/2
  Dot Product58/1 -> Dot Product58_pd1/1
  Dot Product58_pd1/1 -> Out1/1

== system gm_MATE_HDLsolver_myFirstCircuit/ForFPGA/Dot Product59 ==
  In1 : Inport
  In2 : Inport  Port=2
  Dot Product59 : Sum  OutDataTypeStr=single  SampleTime=6.02409638554217e-09
  Dot Product59_pd1 : Delay  DelayLength=6
  Out1 : Outport
  wires:
  In1/1 -> Dot Product59/1
  In2/1 -> Dot Product59/2
  Dot Product59/1 -> Dot Product59_pd1/1
  Dot Product59_pd1/1 -> Out1/1

== system gm_MATE_HDLsolver_myFirstCircuit/ForFPGA/Dot Product6 ==
  In1 : Inport
  In2 : Inport  Port=2
  Dot Product6 : Sum  OutDataTypeStr=single  SampleTime=6.02409638554217e-09
  Dot Product6_pd1 : Delay  DelayLength=6
  Out1 : Outport
  wires:
  In1/1 -> Dot Product6/1
  In2/1 -> Dot Product6/2
  Dot Product6/1 -> Dot Product6_pd1/1
  Dot Product6_pd1/1 -> Out1/1

== system gm_MATE_HDLsolver_myFirstCircuit/ForFPGA/Dot Product61 ==
  In1 : Inport
  In2 : Inport  Port=2
  Dot Product61 : Sum  OutDataTypeStr=single  SampleTime=6.02409638554217e-09
  Dot Product61_pd1 : Delay  DelayLength=6
  Out1 : Outport
  wires:
  In1/1 -> Dot Product61/1
  In2/1 -> Dot Product61/2
  Dot Product61/1 -> Dot Product61_pd1/1
  Dot Product61_pd1/1 -> Out1/1

== system gm_MATE_HDLsolver_myFirstCircuit/ForFPGA/Dot Product610 ==
  In1 : Inport
  In2 : Inport  Port=2
  Dot Product610 : Sum  OutDataTypeStr=single  SampleTime=6.02409638554217e-09
  Dot Product610_pd1 : Delay  DelayLength=6
  Out1 : Outport
  wires:
  In1/1 -> Dot Product610/1
  In2/1 -> Dot Product610/2
  Dot Product610/1 -> Dot Product610_pd1/1
  Dot Product610_pd1/1 -> Out1/1

== system gm_MATE_HDLsolver_myFirstCircuit/ForFPGA/Dot Product611 ==
  In1 : Inport
  In2 : Inport  Port=2
  Dot Product611 : Sum  OutDataTypeStr=single  SampleTime=6.02409638554217e-09
  Dot Product611_pd1 : Delay  DelayLength=6
  Out1 : Outport
  wires:
  In1/1 -> Dot Product611/1
  In2/1 -> Dot Product611/2
  Dot Product611/1 -> Dot Product611_pd1/1
  Dot Product611_pd1/1 -> Out1/1

== system gm_MATE_HDLsolver_myFirstCircuit/ForFPGA/Dot Product612 ==
  In1 : Inport
  In2 : Inport  Port=2
  Dot Product612 : Sum  OutDataTypeStr=single  SampleTime=6.02409638554217e-09
  Dot Product612_pd1 : Delay  DelayLength=6
  Out1 : Outport
  wires:
  In1/1 -> Dot Product612/1
  In2/1 -> Dot Product612/2
  Dot Product612/1 -> Dot Product612_pd1/1
  Dot Product612_pd1/1 -> Out1/1

== system gm_MATE_HDLsolver_myFirstCircuit/ForFPGA/Dot Product613 ==
  In1 : Inport
  In2 : Inport  Port=2
  Dot Product613 : Sum  OutDataTypeStr=single  SampleTime=6.02409638554217e-09
  Dot Product613_pd1 : Delay  DelayLength=6
  Out1 : Outport
  wires:
  In1/1 -> Dot Product613/1
  In2/1 -> Dot Product613/2
  Dot Product613/1 -> Dot Product613_pd1/1
  Dot Product613_pd1/1 -> Out1/1

== system gm_MATE_HDLsolver_myFirstCircuit/ForFPGA/Dot Product614 ==
  In1 : Inport
  In2 : Inport  Port=2
  Dot Product614 : Sum  OutDataTypeStr=single  SampleTime=6.02409638554217e-09
  Dot Product614_pd1 : Delay  DelayLength=6
  Out1 : Outport
  wires:
  In1/1 -> Dot Product614/1
  In2/1 -> Dot Product614/2
  Dot Product614/1 -> Dot Product614_pd1/1
  Dot Product614_pd1/1 -> Out1/1

== system gm_MATE_HDLsolver_myFirstCircuit/ForFPGA/Dot Product615 ==
  In1 : Inport
  In2 : Inport  Port=2
  Dot Product615 : Sum  OutDataTypeStr=single  SampleTime=6.02409638554217e-09
  Dot Product615_pd1 : Delay  DelayLength=6
  Out1 : Outport
  wires:
  In1/1 -> Dot Product615/1
  In2/1 -> Dot Product615/2
  Dot Product615/1 -> Dot Product615_pd1/1
  Dot Product615_pd1/1 -> Out1/1

== system gm_MATE_HDLsolver_myFirstCircuit/ForFPGA/Dot Product62 ==
  In1 : Inport
  In2 : Inport  Port=2
  Dot Product62 : Sum  OutDataTypeStr=single  SampleTime=6.02409638554217e-09
  Dot Product62_pd1 : Delay  DelayLength=6
  Out1 : Outport
  wires:
  In1/1 -> Dot Product62/1
  In2/1 -> Dot Product62/2
  Dot Product62/1 -> Dot Product62_pd1/1
  Dot Product62_pd1/1 -> Out1/1

== system gm_MATE_HDLsolver_myFirstCircuit/ForFPGA/Dot Product63 ==
  In1 : Inport
  In2 : Inport  Port=2
  Dot Product63 : Sum  OutDataTypeStr=single  SampleTime=6.02409638554217e-09
  Dot Product63_pd1 : Delay  DelayLength=6
  Out1 : Outport
  wires:
  In1/1 -> Dot Product63/1
  In2/1 -> Dot Product63/2
  Dot Product63/1 -> Dot Product63_pd1/1
  Dot Product63_pd1/1 -> Out1/1

== system gm_MATE_HDLsolver_myFirstCircuit/ForFPGA/Dot Product64 ==
  In1 : Inport
  In2 : Inport  Port=2
  Dot Product64 : Sum  OutDataTypeStr=single  SampleTime=6.02409638554217e-09
  Dot Product64_pd1 : Delay  DelayLength=6
  Out1 : Outport
  wires:
  In1/1 -> Dot Product64/1
  In2/1 -> Dot Product64/2
  Dot Product64/1 -> Dot Product64_pd1/1
  Dot Product64_pd1/1 -> Out1/1

== system gm_MATE_HDLsolver_myFirstCircuit/ForFPGA/Dot Product65 ==
  In1 : Inport
  In2 : Inport  Port=2
  Dot Product65 : Sum  OutDataTypeStr=single  SampleTime=6.02409638554217e-09
  Dot Product65_pd1 : Delay  DelayLength=6
  Out1 : Outport
  wires:
  In1/1 -> Dot Product65/1
  In2/1 -> Dot Product65/2
  Dot Product65/1 -> Dot Product65_pd1/1
  Dot Product65_pd1/1 -> Out1/1

== system gm_MATE_HDLsolver_myFirstCircuit/ForFPGA/Dot Product66 ==
  In1 : Inport
  In2 : Inport  Port=2
  Dot Product66 : Sum  OutDataTypeStr=single  SampleTime=6.02409638554217e-09
  Dot Product66_pd1 : Delay  DelayLength=6
  Out1 : Outport
  wires:
  In1/1 -> Dot Product66/1
  In2/1 -> Dot Product66/2
  Dot Product66/1 -> Dot Product66_pd1/1
  Dot Product66_pd1/1 -> Out1/1

== system gm_MATE_HDLsolver_myFirstCircuit/ForFPGA/Dot Product67 ==
  In1 : Inport
  In2 : Inport  Port=2
  Dot Product67 : Sum  OutDataTypeStr=single  SampleTime=6.02409638554217e-09
  Dot Product67_pd1 : Delay  DelayLength=6
  Out1 : Outport
  wires:
  In1/1 -> Dot Product67/1
  In2/1 -> Dot Product67/2
  Dot Product67/1 -> Dot Product67_pd1/1
  Dot Product67_pd1/1 -> Out1/1

== system gm_MATE_HDLsolver_myFirstCircuit/ForFPGA/Dot Product68 ==
  In1 : Inport
  In2 : Inport  Port=2
  Dot Product68 : Sum  OutDataTypeStr=single  SampleTime=6.02409638554217e-09
  Dot Product68_pd1 : Delay  DelayLength=6
  Out1 : Outport
  wires:
  In1/1 -> Dot Product68/1
  In2/1 -> Dot Product68/2
  Dot Product68/1 -> Dot Product68_pd1/1
  Dot Product68_pd1/1 -> Out1/1

== system gm_MATE_HDLsolver_myFirstCircuit/ForFPGA/Dot Product69 ==
  In1 : Inport
  In2 : Inport  Port=2
  Dot Product69 : Sum  OutDataTypeStr=single  SampleTime=6.02409638554217e-09
  Dot Product69_pd1 : Delay  DelayLength=6
  Out1 : Outport
  wires:
  In1/1 -> Dot Product69/1
  In2/1 -> Dot Product69/2
  Dot Product69/1 -> Dot Product69_pd1/1
  Dot Product69_pd1/1 -> Out1/1

== system gm_MATE_HDLsolver_myFirstCircuit/ForFPGA/Dot Product7 ==
  In1 : Inport
  In2 : Inport  Port=2
  Dot Product7 : Sum  OutDataTypeStr=single  SampleTime=6.02409638554217e-09
  Dot Product7_pd1 : Delay  DelayLength=6
  Out1 : Outport
  wires:
  In1/1 -> Dot Product7/1
  In2/1 -> Dot Product7/2
  Dot Product7/1 -> Dot Product7_pd1/1
  Dot Product7_pd1/1 -> Out1/1

== system gm_MATE_HDLsolver_myFirstCircuit/ForFPGA/Dot Product71 ==
  In1 : Inport
  In2 : Inport  Port=2
  Dot Product71 : Sum  OutDataTypeStr=single  SampleTime=6.02409638554217e-09
  Dot Product71_pd1 : Delay  DelayLength=6
  Out1 : Outport
  wires:
  In1/1 -> Dot Product71/1
  In2/1 -> Dot Product71/2
  Dot Product71/1 -> Dot Product71_pd1/1
  Dot Product71_pd1/1 -> Out1/1

== system gm_MATE_HDLsolver_myFirstCircuit/ForFPGA/Dot Product710 ==
  In1 : Inport
  In2 : Inport  Port=2
  Dot Product710 : Sum  OutDataTypeStr=single  SampleTime=6.02409638554217e-09
  Dot Product710_pd1 : Delay  DelayLength=6
  Out1 : Outport
  wires:
  In1/1 -> Dot Product710/1
  In2/1 -> Dot Product710/2
  Dot Product710/1 -> Dot Product710_pd1/1
  Dot Product710_pd1/1 -> Out1/1

== system gm_MATE_HDLsolver_myFirstCircuit/ForFPGA/Dot Product711 ==
  In1 : Inport
  In2 : Inport  Port=2
  Dot Product711 : Sum  OutDataTypeStr=single  SampleTime=6.02409638554217e-09
  Dot Product711_pd1 : Delay  DelayLength=6
  Out1 : Outport
  wires:
  In1/1 -> Dot Product711/1
  In2/1 -> Dot Product711/2
  Dot Product711/1 -> Dot Product711_pd1/1
  Dot Product711_pd1/1 -> Out1/1

== system gm_MATE_HDLsolver_myFirstCircuit/ForFPGA/Dot Product712 ==
  In1 : Inport
  In2 : Inport  Port=2
  Dot Product712 : Sum  OutDataTypeStr=single  SampleTime=6.02409638554217e-09
  Dot Product712_pd1 : Delay  DelayLength=6
  Out1 : Outport
  wires:
  In1/1 -> Dot Product712/1
  In2/1 -> Dot Product712/2
  Dot Product712/1 -> Dot Product712_pd1/1
  Dot Product712_pd1/1 -> Out1/1

== system gm_MATE_HDLsolver_myFirstCircuit/ForFPGA/Dot Product713 ==
  In1 : Inport
  In2 : Inport  Port=2
  Dot Product713 : Sum  OutDataTypeStr=single  SampleTime=6.02409638554217e-09
  Dot Product713_pd1 : Delay  DelayLength=6
  Out1 : Outport
  wires:
  In1/1 -> Dot Product713/1
  In2/1 -> Dot Product713/2
  Dot Product713/1 -> Dot Product713_pd1/1
  Dot Product713_pd1/1 -> Out1/1

== system gm_MATE_HDLsolver_myFirstCircuit/ForFPGA/Dot Product714 ==
  In1 : Inport
  In2 : Inport  Port=2
  Dot Product714 : Sum  OutDataTypeStr=single  SampleTime=6.02409638554217e-09
  Dot Product714_pd1 : Delay  DelayLength=6
  Out1 : Outport
  wires:
  In1/1 -> Dot Product714/1
  In2/1 -> Dot Product714/2
  Dot Product714/1 -> Dot Product714_pd1/1
  Dot Product714_pd1/1 -> Out1/1

== system gm_MATE_HDLsolver_myFirstCircuit/ForFPGA/Dot Product715 ==
  In1 : Inport
  In2 : Inport  Port=2
  Dot Product715 : Sum  OutDataTypeStr=single  SampleTime=6.02409638554217e-09
  Dot Product715_pd1 : Delay  DelayLength=6
  Out1 : Outport
  wires:
  In1/1 -> Dot Product715/1
  In2/1 -> Dot Product715/2
  Dot Product715/1 -> Dot Product715_pd1/1
  Dot Product715_pd1/1 -> Out1/1

== system gm_MATE_HDLsolver_myFirstCircuit/ForFPGA/Dot Product72 ==
  In1 : Inport
  In2 : Inport  Port=2
  Dot Product72 : Sum  OutDataTypeStr=single  SampleTime=6.02409638554217e-09
  Dot Product72_pd1 : Delay  DelayLength=6
  Out1 : Outport
  wires:
  In1/1 -> Dot Product72/1
  In2/1 -> Dot Product72/2
  Dot Product72/1 -> Dot Product72_pd1/1
  Dot Product72_pd1/1 -> Out1/1

== system gm_MATE_HDLsolver_myFirstCircuit/ForFPGA/Dot Product73 ==
  In1 : Inport
  In2 : Inport  Port=2
  Dot Product73 : Sum  OutDataTypeStr=single  SampleTime=6.02409638554217e-09
  Dot Product73_pd1 : Delay  DelayLength=6
  Out1 : Outport
  wires:
  In1/1 -> Dot Product73/1
  In2/1 -> Dot Product73/2
  Dot Product73/1 -> Dot Product73_pd1/1
  Dot Product73_pd1/1 -> Out1/1

== system gm_MATE_HDLsolver_myFirstCircuit/ForFPGA/Dot Product74 ==
  In1 : Inport
  In2 : Inport  Port=2
  Dot Product74 : Sum  OutDataTypeStr=single  SampleTime=6.02409638554217e-09
  Dot Product74_pd1 : Delay  DelayLength=6
  Out1 : Outport
  wires:
  In1/1 -> Dot Product74/1
  In2/1 -> Dot Product74/2
  Dot Product74/1 -> Dot Product74_pd1/1
  Dot Product74_pd1/1 -> Out1/1

== system gm_MATE_HDLsolver_myFirstCircuit/ForFPGA/Dot Product75 ==
  In1 : Inport
  In2 : Inport  Port=2
  Dot Product75 : Sum  OutDataTypeStr=single  SampleTime=6.02409638554217e-09
  Dot Product75_pd1 : Delay  DelayLength=6
  Out1 : Outport
  wires:
  In1/1 -> Dot Product75/1
  In2/1 -> Dot Product75/2
  Dot Product75/1 -> Dot Product75_pd1/1
  Dot Product75_pd1/1 -> Out1/1

== system gm_MATE_HDLsolver_myFirstCircuit/ForFPGA/Dot Product76 ==
  In1 : Inport
  In2 : Inport  Port=2
  Dot Product76 : Sum  OutDataTypeStr=single  SampleTime=6.02409638554217e-09
  Dot Product76_pd1 : Delay  DelayLength=6
  Out1 : Outport
  wires:
  In1/1 -> Dot Product76/1
  In2/1 -> Dot Product76/2
  Dot Product76/1 -> Dot Product76_pd1/1
  Dot Product76_pd1/1 -> Out1/1

== system gm_MATE_HDLsolver_myFirstCircuit/ForFPGA/Dot Product77 ==
  In1 : Inport
  In2 : Inport  Port=2
  Dot Product77 : Sum  OutDataTypeStr=single  SampleTime=6.02409638554217e-09
  Dot Product77_pd1 : Delay  DelayLength=6
  Out1 : Outport
  wires:
  In1/1 -> Dot Product77/1
  In2/1 -> Dot Product77/2
  Dot Product77/1 -> Dot Product77_pd1/1
  Dot Product77_pd1/1 -> Out1/1

== system gm_MATE_HDLsolver_myFirstCircuit/ForFPGA/Dot Product78 ==
  In1 : Inport
  In2 : Inport  Port=2
  Dot Product78 : Sum  OutDataTypeStr=single  SampleTime=6.02409638554217e-09
  Dot Product78_pd1 : Delay  DelayLength=6
  Out1 : Outport
  wires:
  In1/1 -> Dot Product78/1
  In2/1 -> Dot Product78/2
  Dot Product78/1 -> Dot Product78_pd1/1
  Dot Product78_pd1/1 -> Out1/1
